simulink model "case12_simulink"  (R2015b)
settings: Solver=VariableStepAuto  StartTime=0.0  StopTime=10.0  RelTol=1e-3
values from neighbouring files (symbols this model uses):
  b = 0.001:.002:.02    [Num4s.m]    (also in cont.m = 0.001:0.002:0.04; lab2case1.m = 2*zeta*wn*.1389*x^2; lab2case1change.m = 2*zeta*wn*.1389*x^2; num2.m = 0.002:0.0008:0.04)
settings Model: Creator=guilh_000  LastModifiedBy=guilh_000

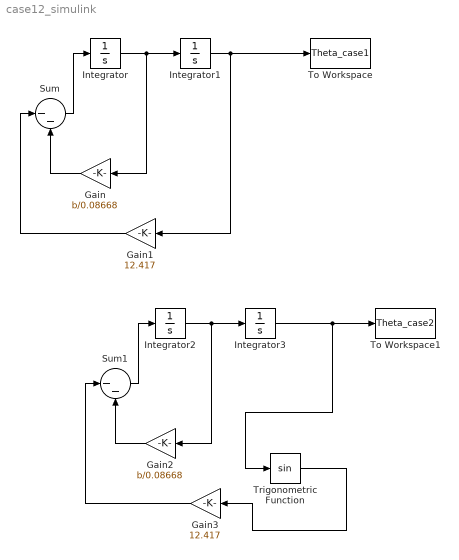
== system case12_simulink ==
  Gain : Gain  Gain=b/0.08668
  Gain1 : Gain  Gain=12.417
  Gain2 : Gain  Gain=b/0.08668
  Gain3 : Gain  Gain=12.417
  Integrator : Integrator
  Integrator1 : Integrator  InitialCondition=pi/4
  Integrator2 : Integrator
  Integrator3 : Integrator  InitialCondition=pi/4
  Sum : Sum  Inputs=|--
  Sum1 : Sum  Inputs=|--
  To Workspace : ToWorkspace  VariableName=Theta_case1  SampleTime=-1
  To Workspace1 : ToWorkspace  VariableName=Theta_case2  SampleTime=-1
  Trigonometric Function : Trigonometry
  wires:
  Integrator/1 -> Gain/1, Integrator1/1
  Sum/1 -> Integrator/1
  Gain/1 -> Sum/2
  Gain1/1 -> Sum/1
  Integrator1/1 -> To Workspace/1, Gain1/1
  Integrator2/1 -> Gain2/1, Integrator3/1
  Sum1/1 -> Integrator2/1
  Gain2/1 -> Sum1/2
  Gain3/1 -> Sum1/1
  Integrator3/1 -> Trigonometric Function/1, To Workspace1/1
  Trigonometric Function/1 -> Gain3/1
